simulink model "eq_2_cond_sim"  (R2021a)
settings: Solver=VariableStepAuto  StartTime=0.0  StopTime=10.0  RelTol=1e-3
settings Model: Creator=55189  LastModifiedBy=55189

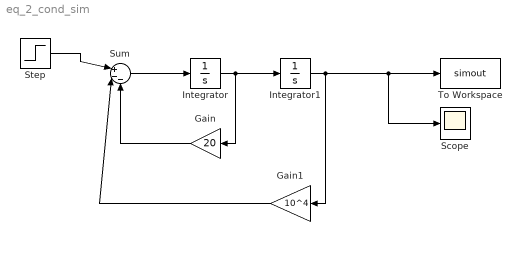
== system eq_2_cond_sim ==
  Gain : Gain  Gain=20
  Gain1 : Gain  Gain=10^4
  Integrator : Integrator  InitialCondition=1
  Integrator1 : Integrator
  Scope : Scope
  Step : Step  Time=0  SampleTime=0
  Sum : Sum  Inputs=|+--
  To Workspace : ToWorkspace  VariableName=simout  SampleTime=-1
  wires:
  Integrator/1 -> Gain/1, Integrator1/1
  Integrator1/1 -> Gain1/1, Scope/1, To Workspace/1
  Sum/1 -> Integrator/1
  Gain/1 -> Sum/3
  Step/1 -> Sum/1
  Gain1/1 -> Sum/2
